simulink model "mag_pd_control_test_new"  (R2016b)
settings: Solver=VariableStepAuto  StartTime=0.0  StopTime=25000  RelTol=1e-3
values from neighbouring files (symbols this model uses):
  omega_cmd = zeros(3,1)    [mag_pd_control_IC_test.m]    (also in mag_pd_control_gain_test_init.m; mag_pd_control_test_init.m)
  quat_cmd = [1;0;0;0]    [mag_pd_control_IC_test.m]    (also in mag_pd_control_gain_test_init.m; mag_pd_control_test_init.m)
libraries: dynamics_lib x1, environment_lib x1, aerolibutil x1, bus_stubs_template x1, mag_PD_control_new x1, magnetorquer_assembly_lib x1
settings Model: Creator=bijan  LastModifiedBy=bijan

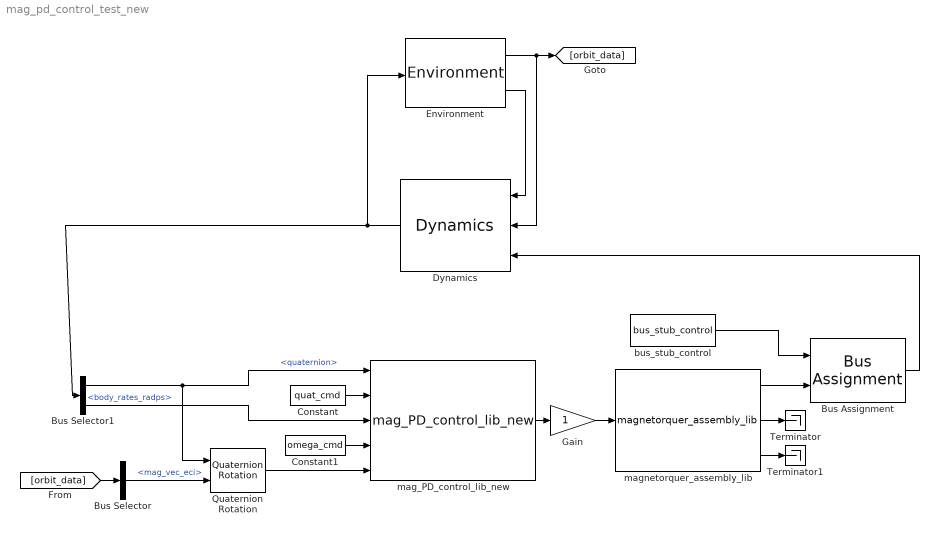
== system mag_pd_control_test_new ==
  Bus Assignment : BusAssignment  AssignedSignals=MT_dipole_Am2
  Bus Selector : BusSelector  OutputSignals=mag_vec_eci
  Bus Selector1 : BusSelector  OutputSignals=quaternion,body_rates_radps
  Constant : Constant  Value=quat_cmd
  Constant1 : Constant  Value=omega_cmd
  Dynamics : dynamics_lib/Dynamics
  Environment : environment_lib/Environment
  Gain : Gain
  Quaternion Rotation : aerolibutil/Quaternion Rotation
  Terminator : Terminator
  Terminator1 : Terminator
  bus_stub_control : bus_stubs_template/bus_stub_control
  "mag_PD_control_lib_new " : mag_PD_control_new/mag_PD_control_lib_new 
  magnetorquer_assembly_lib : magnetorquer_assembly_lib/magnetorquer_assembly_lib
  wires:
  Environment/2 -> Dynamics/1
  Environment/1 -> [orbit_data], Dynamics/2
  Dynamics/1 -> Environment/1, Bus Selector1/1
  "mag_PD_control_lib_new "/1 -> Gain/1
  Constant/1 -> "mag_PD_control_lib_new "/2
  Constant1/1 -> "mag_PD_control_lib_new "/4
  [orbit_data] -> Bus Selector/1
  Bus Selector/1 -> Quaternion Rotation/2  "<mag_vec_eci>"
  Bus Selector1/1 -> "mag_PD_control_lib_new "/1, Quaternion Rotation/1  "<quaternion>"
  Bus Selector1/2 -> "mag_PD_control_lib_new "/3  "<body_rates_radps>"
  Quaternion Rotation/1 -> "mag_PD_control_lib_new "/5
  bus_stub_control/1 -> Bus Assignment/1
  magnetorquer_assembly_lib/1 -> Bus Assignment/2
  magnetorquer_assembly_lib/2 -> Terminator/1
  magnetorquer_assembly_lib/3 -> Terminator1/1
  Bus Assignment/1 -> Dynamics/3
  Gain/1 -> magnetorquer_assembly_lib/1
